simulink library "acolibjan22"  (R2021a)
settings: Solver=VariableStepAuto  StartTime=0.0  StopTime=10.0  RelTol=1e-3
libraries: simulink_extras x5, simulink x2, $bdroot x2
settings Model: Creator=e102261  LastModifiedBy=e102261
settings SolverCC: AlgebraicLoopSolver=TrustRegion
settings DebuggingCC: ArithmeticOperatorsInVariantConditions=warning
settings SFSimCC: CustomCodeUndefinedFunction=UseInterfaceOnly

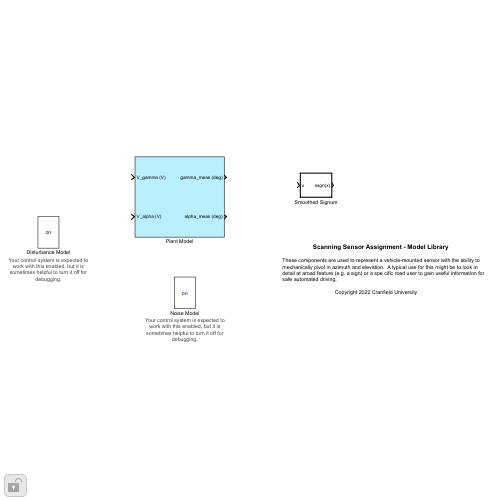
[thumbnail: Simulink's stored preview of the top-level diagram]
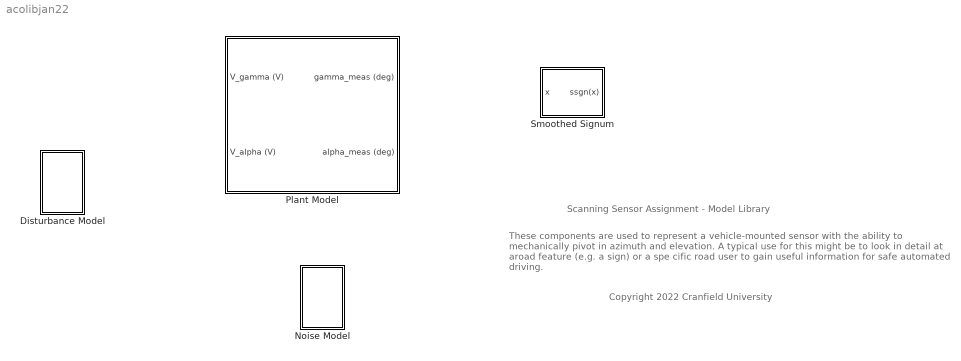
== system acolibjan22 ==
  note: Copyright 2022 Cranfield University
  note: Scanning Sensor Assignment - Model Library
  note: These components are used to represent a vehicle-mounted sensor with the ability to mechanically pivot in azimuth and elevation.  A typical use for this might be to look in
      | detail at aroad feature (e.g. a sign) or a spe cific road user to gain useful information for
      | safe automated driving.
  Disturbance Model : Subsystem  mask(Disturbance Model){EnabledState=on}
      mask prompts: EnabledState "Enable"
      mask help: This block implements a disturbance model.
      mask init:
      | if EnabledState
      |     theText = 'on';
      |     theColor = 'blue';
      | else
      |     theText = 'off';
      |     theColor = 'red';
      | end
      settings: AttributesFormatString=|
      | Your control system is expected to
      | work with this enabled, but it is
      | sometimes helpful to turn it off for
      | debugging.
      mask Display:
      | color(theColor);
      | fprintf(theText);
  Noise Model : Subsystem  mask(Noise Model){EnabledState=on}
      mask prompts: EnabledState "Enable"
      mask help: This block implements a noise model.
      mask init:
      | if EnabledState
      |     theText = 'on';
      |     theColor = 'blue';
      | else
      |     theText = 'off';
      |     theColor = 'red';
      | end
      settings: AttributesFormatString=|
      | Your control system is expected to
      | work with this enabled, but it is
      | sometimes helpful to turn it off for
      | debugging.
      mask Display:
      | color(theColor);
      | fprintf(theText);
  Plant Model : Subsystem  mask{X0=0}
      mask prompts: X0 "Initial state:"
      mask init:
      | if isequal(X0, 0)
      |     X0 = zeros(6,1);
      | else
      |     X0 = [X0(1); X0(2); X0(3); X0(4); X0(5); X0(6)];
      | end
  Smoothed Signum : Subsystem  TreatAsAtomicUnit=on  mask(Smoothed Signum){ApproxTransitionBand=0.1}
      mask prompts: ApproxTransitionBand "Approx. transition band (units):"
      mask help: This block implements a smoothed signum function, suitable for modelling stuff like friction. This can make it easier to implement near-hybrid models that execute nicely.
      mask init:
      | G = 1 / double(ApproxTransitionBand(1));

== system acolibjan22/Disturbance Model ==
  Constant : Constant  Value=EnabledState
  Enabled Subsystem : Subsystem
  tag scope: daz=global, del=global
  wires:
  Enabled Subsystem/1(daz) -> [daz]
  Enabled Subsystem/2(del) -> [del]
  Constant/1 -> Enabled Subsystem/Enable

== system acolibjan22/Noise Model ==
  Constant : Constant  Value=EnabledState
  Enabled Subsystem : Subsystem
  tag scope: waz=global, wel=global
  wires:
  Constant/1 -> Enabled Subsystem/Enable
  Enabled Subsystem/2(wel) -> [wel]
  Enabled Subsystem/1(waz) -> [waz]

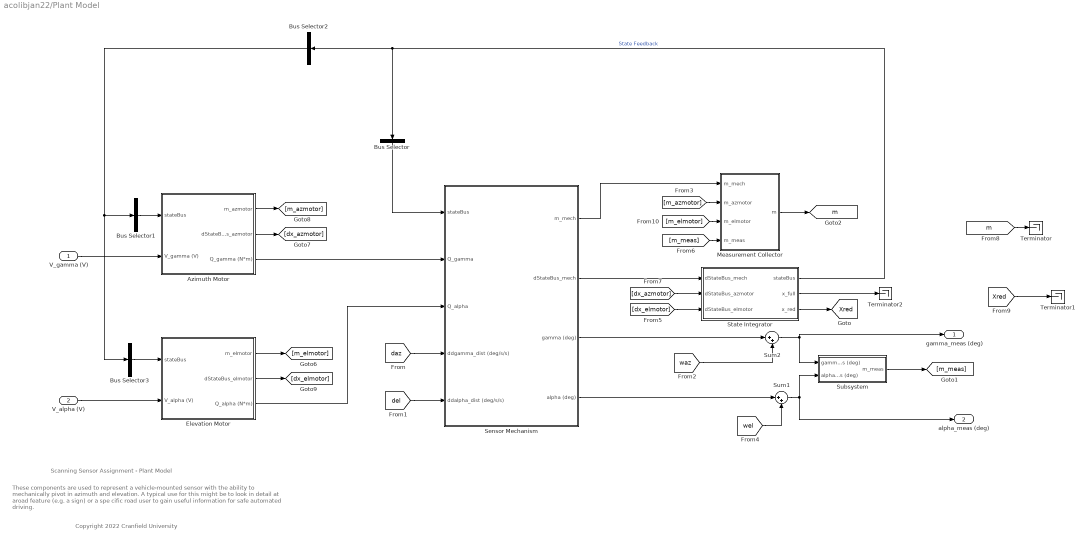
== system acolibjan22/Plant Model ==
  note: These components are used to represent a vehicle-mounted sensor with the ability to mechanically pivot in azimuth and elevation.  A typical use for this might be to look in
      | detail at aroad feature (e.g. a sign) or a spe cific road user to gain useful information for
      | safe automated driving.
  note: Scanning Sensor Assignment - Plant Model
  note: Copyright 2022 Cranfield University
  V_gamma (V) : Inport
  V_alpha (V) : Inport  Port=2
  Azimuth Motor : Subsystem
  Bus Selector : BusSelector  OutputSignals=gamma,dgamma,alpha,dalpha  OutputAsBus=on
  Bus Selector1 : BusSelector  OutputSignals=Q_gamma  OutputAsBus=on
  Bus Selector2 : BusSelector  OutputSignals=Q_gamma,Q_alpha  OutputAsBus=on
  Bus Selector3 : BusSelector  OutputSignals=Q_alpha  OutputAsBus=on
  Elevation Motor : Subsystem
  Measurement Collector : Subsystem
  Sensor Mechanism : Subsystem
  State Integrator : Subsystem
  Subsystem : Subsystem
  Sum1 : Sum  Inputs=|++
  Sum2 : Sum  Inputs=|++
  Terminator : Terminator
  Terminator1 : Terminator
  Terminator2 : Terminator
  gamma_meas (deg) : Outport
  alpha_meas (deg) : Outport  Port=2
  tag scope: Xred=global, m=global
  wires:
  [Xred] -> Terminator1/1
  Sensor Mechanism/4(alpha (deg)) -> Sum1/1
  Azimuth Motor/3(Q_gamma (N*m)) -> Sensor Mechanism/2(Q_gamma)
  V_gamma (V)/1 -> Azimuth Motor/2(V_gamma (V))
  [daz] -> Sensor Mechanism/4(ddgamma_dist (deg/s/s))
  [del] -> Sensor Mechanism/5(ddalpha_dist (deg/s/s))
  V_alpha (V)/1 -> Elevation Motor/2(V_alpha (V))
  State Integrator/1(stateBus) -> Bus Selector/1, Bus Selector2/1  "State Feedback"
  Azimuth Motor/1(m_azmotor) -> [m_azmotor]
  Measurement Collector/1(m) -> [m]
  [m_azmotor] -> Measurement Collector/2(m_azmotor)
  Azimuth Motor/2(dStateBus_azmotor) -> [dx_azmotor]
  [dx_azmotor] -> State Integrator/2(dStateBus_azmotor)
  Elevation Motor/1(m_elmotor) -> [m_elmotor]
  Elevation Motor/2(dStateBus_elmotor) -> [dx_elmotor]
  Elevation Motor/3(Q_alpha (N*m)) -> Sensor Mechanism/3(Q_alpha)
  [dx_elmotor] -> State Integrator/3(dStateBus_elmotor)
  [m_elmotor] -> Measurement Collector/3(m_elmotor)
  Sensor Mechanism/2(dStateBus_mech) -> State Integrator/1(dStateBus_mech)
  Sensor Mechanism/1(m_mech) -> Measurement Collector/1(m_mech)
  Bus Selector/1 -> Sensor Mechanism/1(stateBus)
  Bus Selector2/1 -> Bus Selector3/1, Bus Selector1/1
  Bus Selector1/1 -> Azimuth Motor/1(stateBus)
  Bus Selector3/1 -> Elevation Motor/1(stateBus)
  State Integrator/2(x_full) -> Terminator2/1
  State Integrator/3(x_red) -> [Xred]
  Sum1/1 -> Subsystem/2(alpha_meas (deg)), alpha_meas (deg)/1
  [wel] -> Sum1/2
  Sensor Mechanism/3(gamma (deg)) -> Sum2/1
  [waz] -> Sum2/2
  Sum2/1 -> Subsystem/1(gamma_meas (deg)), gamma_meas (deg)/1
  Subsystem/1(m_meas) -> [m_meas]
  [m_meas] -> Measurement Collector/4(m_meas)
  [m] -> Terminator/1

== system acolibjan22/Smoothed Signum ==
  x : Inport  PortDimensions=1
  Abs : Abs
  Product : Product  Inputs=3
  Product1 : Product
  Sign : Signum
  Transition Rate : Gain  Gain=8*G
  Trigonometric Function : Trigonometry  Operator=tanh
  ssgn(x) : Outport  PortDimensions=1
  wires:
  Product1/1 -> ssgn(x)/1
  Transition Rate/1 -> Trigonometric Function/1
  x/1 -> Sign/1, Transition Rate/1
  Trigonometric Function/1 -> Abs/1
  Abs/1 -> Product/3, Product/1, Product/2
  Product/1 -> Product1/1
  Sign/1 -> Product1/2

== system acolibjan22/Disturbance Model/Enabled Subsystem ==
  Enable : EnablePort
  Band-Limited White Noise : simulink/Sources/Band-Limited White Noise  Cov=5^2  Ts=0.8  seed=12414
  Band-Limited White Noise1 : simulink/Sources/Band-Limited White Noise  Cov=5^2  Ts=1.2  seed=43214517
  daz : Outport  OutputWhenDisabled=reset  InitialOutput=0
  del : Outport  Port=2  OutputWhenDisabled=reset  InitialOutput=0
  wires:
  Band-Limited White Noise1/1 -> del/1
  Band-Limited White Noise/1 -> daz/1

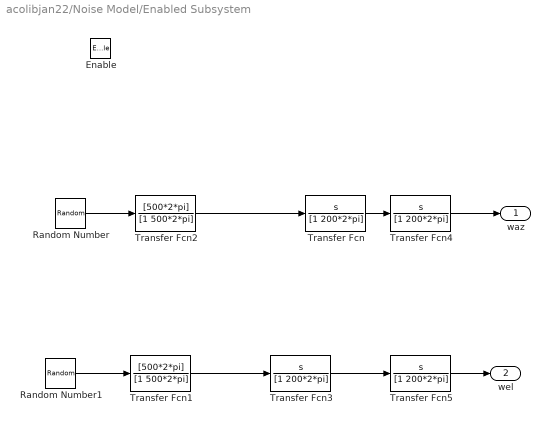
== system acolibjan22/Noise Model/Enabled Subsystem ==
  Enable : EnablePort
  Random Number : RandomNumber  Seed=8576  SampleTime=1/1000
  Random Number1 : RandomNumber  Seed=325325  SampleTime=1/500
  Transfer Fcn{,3..5} (4 alike) : TransferFcn  Numerator=[1 0]  Denominator=[1 200*2*pi]
  Transfer Fcn1 : TransferFcn  Numerator=[500*2*pi]  Denominator=[1 500*2*pi]
  Transfer Fcn2 : TransferFcn  Numerator=[500*2*pi]  Denominator=[1 500*2*pi]
  waz : Outport  OutputWhenDisabled=reset  InitialOutput=0
  wel : Outport  Port=2  OutputWhenDisabled=reset  InitialOutput=0
  wires:
  Transfer Fcn5/1 -> wel/1
  Transfer Fcn4/1 -> waz/1
  Transfer Fcn/1 -> Transfer Fcn4/1
  Random Number/1 -> Transfer Fcn2/1
  Transfer Fcn2/1 -> Transfer Fcn/1
  Random Number1/1 -> Transfer Fcn1/1
  Transfer Fcn3/1 -> Transfer Fcn5/1
  Transfer Fcn1/1 -> Transfer Fcn3/1

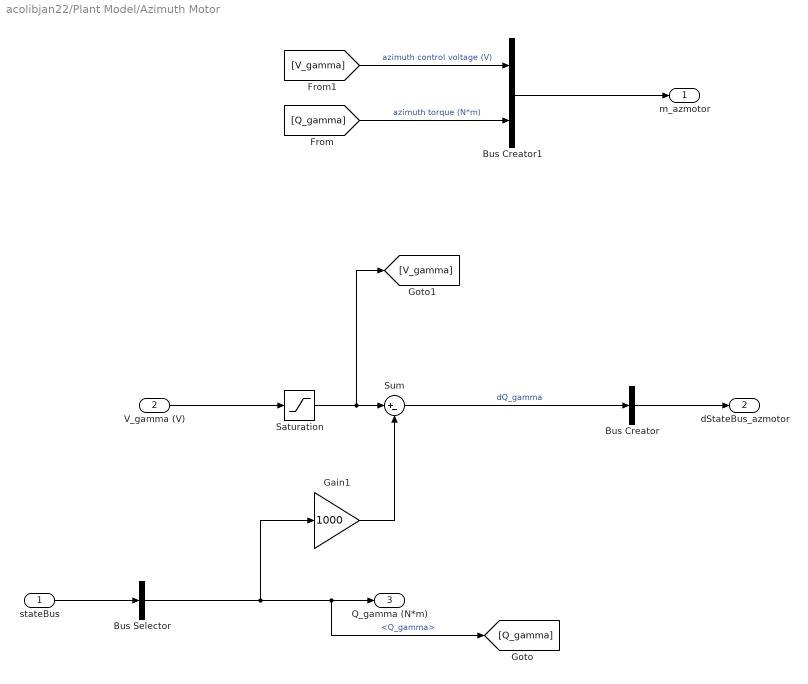
== system acolibjan22/Plant Model/Azimuth Motor ==
  stateBus : Inport
  V_gamma (V) : Inport  Port=2
  Bus Creator : BusCreator  Inputs=1
  Bus Creator1 : BusCreator  Inputs=2
  Bus Selector : BusSelector  OutputSignals=Q_gamma
  Gain1 : Gain  Gain=1000
  Saturation : Saturate  UpperLimit=+15  LowerLimit=-15
      settings: AttributesFormatString=|
      | UpperLimit=%<UpperLimit>
      | LowerLimit=%<LowerLimit>
  Sum : Sum  Inputs=|+-
  m_azmotor : Outport
  dStateBus_azmotor : Outport  Port=2
  Q_gamma (N*m) : Outport  Port=3
  wires:
  Saturation/1 -> [V_gamma], Sum/1
  V_gamma (V)/1 -> Saturation/1
  Gain1/1 -> Sum/2
  Sum/1 -> Bus Creator/1  "dQ_gamma"
  stateBus/1 -> Bus Selector/1
  Bus Selector/1 -> Gain1/1, [Q_gamma], Q_gamma (N*m)/1  "<Q_gamma>"
  Bus Creator/1 -> dStateBus_azmotor/1
  [Q_gamma] -> Bus Creator1/2  "azimuth torque (N*m)"
  [V_gamma] -> Bus Creator1/1  "azimuth control voltage (V)"
  Bus Creator1/1 -> m_azmotor/1

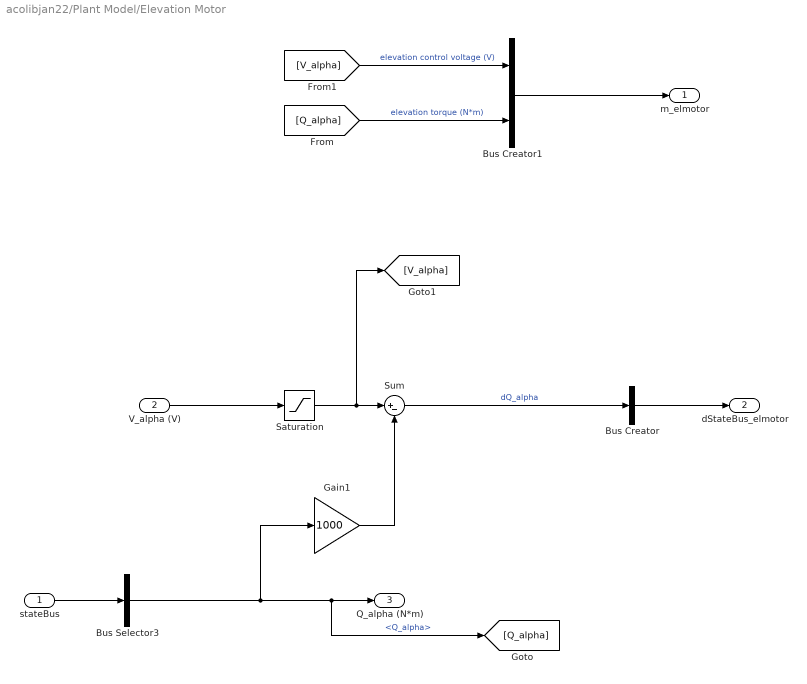
== system acolibjan22/Plant Model/Elevation Motor ==
  stateBus : Inport
  V_alpha (V) : Inport  Port=2
  Bus Creator : BusCreator  Inputs=1
  Bus Creator1 : BusCreator  Inputs=2
  Bus Selector3 : BusSelector  OutputSignals=Q_alpha
  Gain1 : Gain  Gain=1000
  Saturation : Saturate  UpperLimit=+15  LowerLimit=-15
      settings: AttributesFormatString=|
      | UpperLimit=%<UpperLimit>
      | LowerLimit=%<LowerLimit>
  Sum : Sum  Inputs=|+-
  m_elmotor : Outport
  dStateBus_elmotor : Outport  Port=2
  Q_alpha (N*m) : Outport  Port=3
  wires:
  Saturation/1 -> [V_alpha], Sum/1
  V_alpha (V)/1 -> Saturation/1
  Gain1/1 -> Sum/2
  Sum/1 -> Bus Creator/1  "dQ_alpha"
  stateBus/1 -> Bus Selector3/1
  Bus Creator/1 -> dStateBus_elmotor/1
  [Q_alpha] -> Bus Creator1/2  "elevation torque (N*m)"
  [V_alpha] -> Bus Creator1/1  "elevation control voltage (V)"
  Bus Creator1/1 -> m_elmotor/1
  Bus Selector3/1 -> Gain1/1, [Q_alpha], Q_alpha (N*m)/1  "<Q_alpha>"

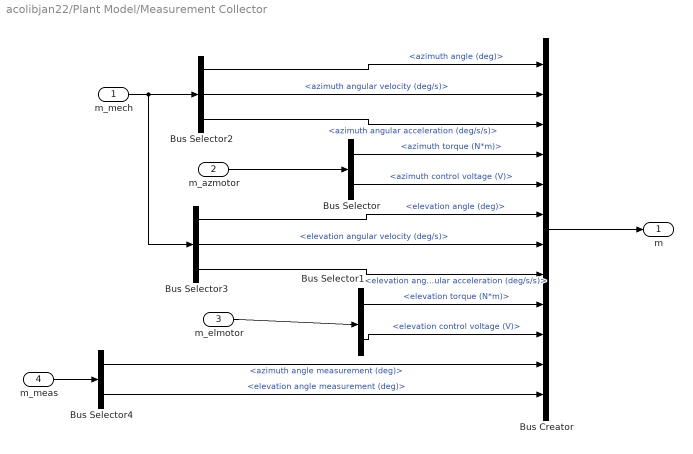
== system acolibjan22/Plant Model/Measurement Collector ==
  m_mech : Inport
  m_azmotor : Inport  Port=2
  m_elmotor : Inport  Port=3
  m_meas : Inport  Port=4
  Bus Creator : BusCreator  Inputs=12
  Bus Selector : BusSelector  OutputSignals=azimuth torque (N*m),azimuth control voltage (V)
  Bus Selector1 : BusSelector  OutputSignals=elevation torque (N*m),elevation control voltage (V)
  Bus Selector2 : BusSelector  OutputSignals=azimuth angle (deg),azimuth angular velocity (deg/s),azimuth angular acceleration (deg/s/s)
  Bus Selector3 : BusSelector  OutputSignals=elevation angle (deg),elevation angular velocity (deg/s),elevation angular acceleration (deg/s/s)
  Bus Selector4 : BusSelector  OutputSignals=azimuth angle measurement (deg),elevation angle measurement (deg)
  m : Outport
  wires:
  Bus Creator/1 -> m/1
  Bus Selector3/1 -> Bus Creator/6  "<elevation angle (deg)>"
  Bus Selector1/2 -> Bus Creator/10  "<elevation control voltage (V)>"
  Bus Selector1/1 -> Bus Creator/9  "<elevation torque (N*m)>"
  Bus Selector3/2 -> Bus Creator/7  "<elevation angular velocity (deg/s)>"
  Bus Selector3/3 -> Bus Creator/8  "<elevation angular acceleration (deg/s/s)>"
  m_azmotor/1 -> Bus Selector/1
  Bus Selector/1 -> Bus Creator/4  "<azimuth torque (N*m)>"
  Bus Selector/2 -> Bus Creator/5  "<azimuth control voltage (V)>"
  m_elmotor/1 -> Bus Selector1/1
  m_mech/1 -> Bus Selector3/1, Bus Selector2/1
  Bus Selector2/1 -> Bus Creator/1  "<azimuth angle (deg)>"
  Bus Selector2/2 -> Bus Creator/2  "<azimuth angular velocity (deg/s)>"
  Bus Selector2/3 -> Bus Creator/3  "<azimuth angular acceleration (deg/s/s)>"
  m_meas/1 -> Bus Selector4/1
  Bus Selector4/1 -> Bus Creator/11  "<azimuth angle measurement (deg)>"
  Bus Selector4/2 -> Bus Creator/12  "<elevation angle measurement (deg)>"

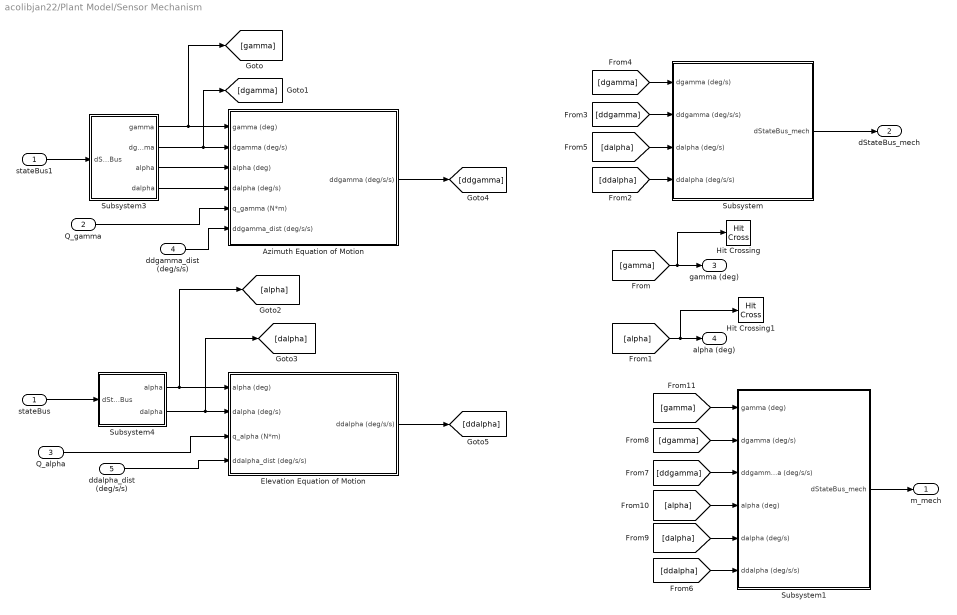
== system acolibjan22/Plant Model/Sensor Mechanism ==
  stateBus : Inport
  Q_gamma : Inport  Port=2
  Q_alpha : Inport  Port=3
  ddgamma_dist (deg/s/s) : Inport  Port=4
  ddalpha_dist (deg/s/s) : Inport  Port=5
  Azimuth Equation of Motion : Subsystem  mask{J=1e-3, Ja=0.020e-3, F=0.1e-3, k=1e-3}
      mask prompts: J "Fixed moment of inertia:"; Ja "Varying moment of inertia:"; F "Coefficient of friction (N*m):"; k "Coefficient of damping (N*m/rad/s):"
  Elevation Equation of Motion : Subsystem  mask(Elevation Dynamics){J=1e-3, F=0.1e-3, k=1e-3}
      mask prompts: J "Moment of inertia"; F "Coefficient of friction (N):"; k "Coefficient of damping (N*m/rad/s):"
      mask help: This block represents the elevantion dynamics of the sensor mount.
  Hit Crossing : HitCross  HitCrossingOffset=linspace(-180,180,361)  ShowOutputPort=off
  Hit Crossing1 : HitCross  HitCrossingOffset=linspace(-180,180,361)  ShowOutputPort=off
  Subsystem : Subsystem
  Subsystem1 : Subsystem
  Subsystem3 : Subsystem
  Subsystem4 : Subsystem
  stateBus1 : InportShadow
  m_mech : Outport
  dStateBus_mech : Outport  Port=2
  gamma (deg) : Outport  Port=3
  alpha (deg) : Outport  Port=4
  wires:
  ddalpha_dist (deg/s/s)/1 -> Elevation Equation of Motion/4(ddalpha_dist (deg/s/s))
  Elevation Equation of Motion/1(ddalpha (deg/s/s)) -> [ddalpha]
  ddgamma_dist (deg/s/s)/1 -> Azimuth Equation of Motion/6(ddgamma_dist (deg/s/s))
  Azimuth Equation of Motion/1(ddgamma (deg/s/s)) -> [ddgamma]
  stateBus1/1 -> Subsystem3/1(dStateBus)
  Q_gamma/1 -> Azimuth Equation of Motion/5(q_gamma (N*m))
  stateBus/1 -> Subsystem4/1(dStateBus)
  Q_alpha/1 -> Elevation Equation of Motion/3(q_alpha (N*m))
  Subsystem3/1(gamma) -> [gamma], Azimuth Equation of Motion/1(gamma (deg))
  Subsystem3/2(dgamma) -> [dgamma], Azimuth Equation of Motion/2(dgamma (deg/s))
  Subsystem3/3(alpha) -> Azimuth Equation of Motion/3(alpha (deg))
  Subsystem3/4(dalpha) -> Azimuth Equation of Motion/4(dalpha (deg/s))
  Subsystem4/1(alpha) -> Elevation Equation of Motion/1(alpha (deg)), [alpha]
  Subsystem4/2(dalpha) -> [dalpha], Elevation Equation of Motion/2(dalpha (deg/s))
  [gamma] -> Hit Crossing/1, gamma (deg)/1
  [alpha] -> Hit Crossing1/1, alpha (deg)/1
  [ddalpha] -> Subsystem/4(ddalpha (deg/s/s))
  [ddgamma] -> Subsystem/2(ddgamma (deg/s/s))
  [dgamma] -> Subsystem/1(dgamma (deg/s))
  [dalpha] -> Subsystem/3(dalpha (deg/s))
  Subsystem/1(dStateBus_mech) -> dStateBus_mech/1
  [ddalpha] -> Subsystem1/6(ddalpha (deg/s/s))
  [dalpha] -> Subsystem1/5(dalpha (deg/s))
  [ddgamma] -> Subsystem1/3(ddgamma (deg/s/s))
  [dgamma] -> Subsystem1/2(dgamma (deg/s))
  [alpha] -> Subsystem1/4(alpha (deg))
  [gamma] -> Subsystem1/1(gamma (deg))
  Subsystem1/1(dStateBus_mech) -> m_mech/1

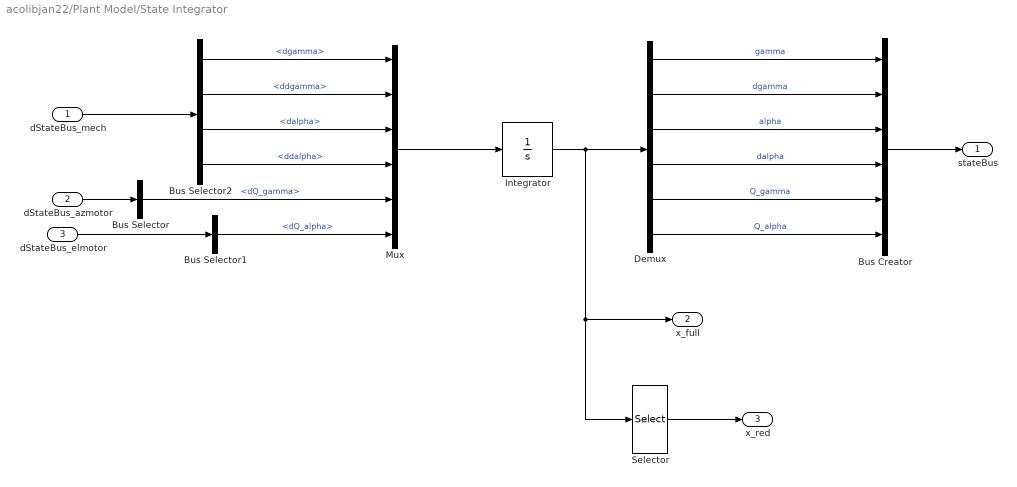
== system acolibjan22/Plant Model/State Integrator ==
  dStateBus_mech : Inport
  dStateBus_azmotor : Inport  Port=2
  dStateBus_elmotor : Inport  Port=3
  Bus Creator : BusCreator  Inputs=6
  Bus Selector : BusSelector  OutputSignals=dQ_gamma
  Bus Selector1 : BusSelector  OutputSignals=dQ_alpha
  Bus Selector2 : BusSelector  OutputSignals=dgamma,ddgamma,dalpha,ddalpha
  Demux : Demux  Outputs=6
  Integrator : Integrator  InitialCondition=X0
  Mux : Mux  Inputs=6
  Selector : Selector  InputPortWidth=6  IndexOptions=Index vector (dialog)  Indices=[1:4]  OutputSizes=1
  stateBus : Outport
  x_full : Outport  Port=2
  x_red : Outport  Port=3
  wires:
  Mux/1 -> Integrator/1
  Bus Selector/1 -> Mux/5  "<dQ_gamma>"
  dStateBus_azmotor/1 -> Bus Selector/1
  dStateBus_elmotor/1 -> Bus Selector1/1
  Bus Selector1/1 -> Mux/6  "<dQ_alpha>"
  dStateBus_mech/1 -> Bus Selector2/1
  Bus Selector2/1 -> Mux/1  "<dgamma>"
  Bus Selector2/2 -> Mux/2  "<ddgamma>"
  Bus Selector2/4 -> Mux/4  "<ddalpha>"
  Bus Selector2/3 -> Mux/3  "<dalpha>"
  Demux/3 -> Bus Creator/3  "alpha"
  Demux/6 -> Bus Creator/6  "Q_alpha"
  Demux/2 -> Bus Creator/2  "dgamma"
  Integrator/1 -> x_full/1, Selector/1, Demux/1
  Bus Creator/1 -> stateBus/1
  Demux/4 -> Bus Creator/4  "dalpha"
  Demux/5 -> Bus Creator/5  "Q_gamma"
  Demux/1 -> Bus Creator/1  "gamma"
  Selector/1 -> x_red/1

== system acolibjan22/Plant Model/Subsystem ==
  gamma_meas (deg) : Inport
  alpha_meas (deg) : Inport  Port=2
  Bus Creator : BusCreator  Inputs=2
  m_meas : Outport
  wires:
  gamma_meas (deg)/1 -> Bus Creator/1  "azimuth angle measurement (deg)"
  alpha_meas (deg)/1 -> Bus Creator/2  "elevation angle measurement (deg)"
  Bus Creator/1 -> m_meas/1

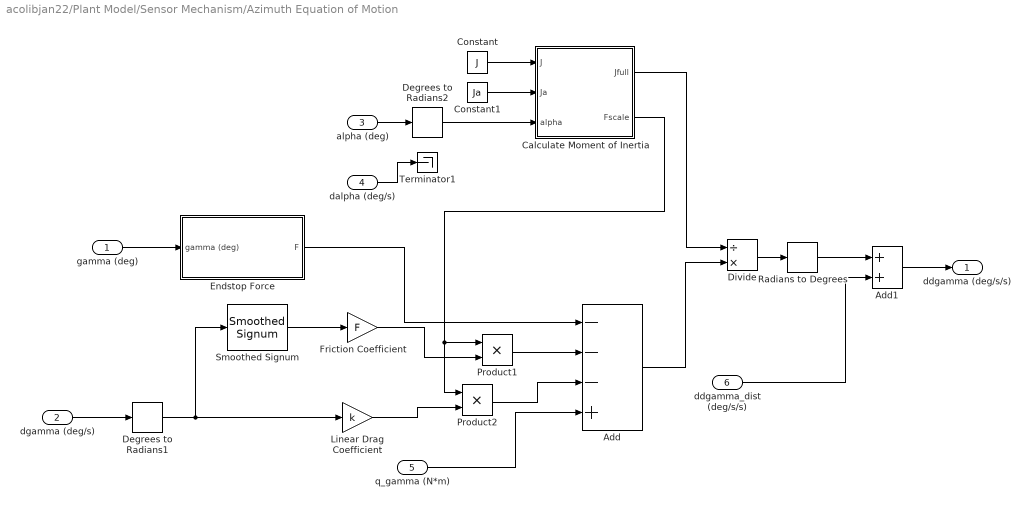
== system acolibjan22/Plant Model/Sensor Mechanism/Azimuth Equation of Motion ==
  gamma (deg) : Inport
  dgamma (deg/s) : Inport  Port=2
  alpha (deg) : Inport  Port=3
  dalpha (deg/s) : Inport  Port=4
  q_gamma (N*m) : Inport  Port=5
  ddgamma_dist (deg/s/s) : Inport  Port=6
  Add : Sum  Inputs=---+
  Add1 : Sum
  Calculate Moment of Inertia : Subsystem
  Constant : Constant  Value=J
  Constant1 : Constant  Value=Ja
  Degrees to Radians1 : simulink_extras/Transformations/Degrees to Radians
  Degrees to Radians2 : simulink_extras/Transformations/Degrees to Radians
  Divide : Product  Inputs=/*
  Endstop Force : Subsystem
  Friction Coefficient : Gain  Gain=F
  Linear Drag Coefficient : Gain  Gain=k
  Product1 : Product
  Product2 : Product
  Radians to Degrees : simulink_extras/Transformations/Radians to Degrees
  Smoothed Signum : $bdroot/Smoothed Signum  ApproxTransitionBand=0.1
  Terminator1 : Terminator
  ddgamma (deg/s/s) : Outport
  wires:
  Product2/1 -> Add/3
  Product1/1 -> Add/2
  Calculate Moment of Inertia/2(Fscale) -> Product2/1, Product1/1
  Radians to Degrees/1 -> Add1/1
  Add1/1 -> ddgamma (deg/s/s)/1
  ddgamma_dist (deg/s/s)/1 -> Add1/2
  Divide/1 -> Radians to Degrees/1
  Add/1 -> Divide/2
  Linear Drag Coefficient/1 -> Product2/2
  q_gamma (N*m)/1 -> Add/4
  Degrees to Radians1/1 -> Smoothed Signum/1, Linear Drag Coefficient/1
  dgamma (deg/s)/1 -> Degrees to Radians1/1
  Friction Coefficient/1 -> Product1/2
  Smoothed Signum/1 -> Friction Coefficient/1
  alpha (deg)/1 -> Degrees to Radians2/1
  Constant/1 -> Calculate Moment of Inertia/1(J)
  Degrees to Radians2/1 -> Calculate Moment of Inertia/3(alpha)
  Constant1/1 -> Calculate Moment of Inertia/2(Ja)
  Calculate Moment of Inertia/1(Jfull) -> Divide/1
  gamma (deg)/1 -> Endstop Force/1(gamma (deg))
  dalpha (deg/s)/1 -> Terminator1/1
  Endstop Force/1(F) -> Add/1

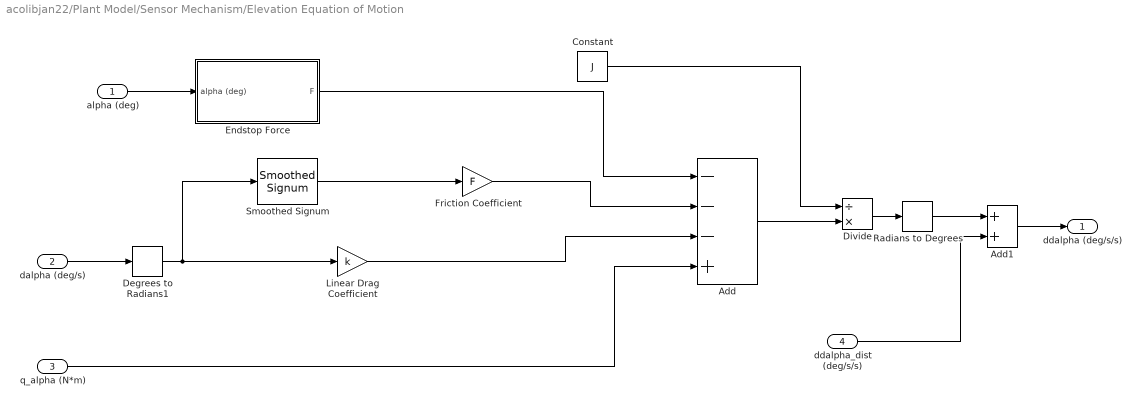
== system acolibjan22/Plant Model/Sensor Mechanism/Elevation Equation of Motion ==
  alpha (deg) : Inport
  dalpha (deg/s) : Inport  Port=2
  q_alpha (N*m) : Inport  Port=3
  ddalpha_dist (deg/s/s) : Inport  Port=4
  Add : Sum  Inputs=---+
  Add1 : Sum
  Constant : Constant  Value=J
  Degrees to Radians1 : simulink_extras/Transformations/Degrees to Radians
  Divide : Product  Inputs=/*
  Endstop Force : Subsystem
  Friction Coefficient : Gain  Gain=F
  Linear Drag Coefficient : Gain  Gain=k
  Radians to Degrees : simulink_extras/Transformations/Radians to Degrees
  Smoothed Signum : $bdroot/Smoothed Signum  ApproxTransitionBand=0.1
  ddalpha (deg/s/s) : Outport
  wires:
  Smoothed Signum/1 -> Friction Coefficient/1
  Friction Coefficient/1 -> Add/2
  dalpha (deg/s)/1 -> Degrees to Radians1/1
  Degrees to Radians1/1 -> Linear Drag Coefficient/1, Smoothed Signum/1
  q_alpha (N*m)/1 -> Add/4
  Linear Drag Coefficient/1 -> Add/3
  Add/1 -> Divide/2
  Divide/1 -> Radians to Degrees/1
  ddalpha_dist (deg/s/s)/1 -> Add1/2
  Add1/1 -> ddalpha (deg/s/s)/1
  Radians to Degrees/1 -> Add1/1
  Constant/1 -> Divide/1
  alpha (deg)/1 -> Endstop Force/1(alpha (deg))
  Endstop Force/1(F) -> Add/1

== system acolibjan22/Plant Model/Sensor Mechanism/Subsystem ==
  dgamma (deg/s) : Inport
  ddgamma (deg/s/s) : Inport  Port=2
  dalpha (deg/s) : Inport  Port=3
  ddalpha (deg/s/s) : Inport  Port=4
  Bus Creator : BusCreator  Inputs=4
  dStateBus_mech : Outport
  wires:
  ddgamma (deg/s/s)/1 -> Bus Creator/2  "ddgamma"
  dgamma (deg/s)/1 -> Bus Creator/1  "dgamma"
  Bus Creator/1 -> dStateBus_mech/1
  ddalpha (deg/s/s)/1 -> Bus Creator/4  "ddalpha"
  dalpha (deg/s)/1 -> Bus Creator/3  "dalpha"

== system acolibjan22/Plant Model/Sensor Mechanism/Subsystem1 ==
  gamma (deg) : Inport
  dgamma (deg/s) : Inport  Port=2
  ddgamma (deg/s/s) : Inport  Port=3
  alpha (deg) : Inport  Port=4
  dalpha (deg/s) : Inport  Port=5
  ddalpha (deg/s/s) : Inport  Port=6
  Bus Creator : BusCreator  Inputs=6
  dStateBus_mech : Outport
  wires:
  dalpha (deg/s)/1 -> Bus Creator/5  "elevation angular velocity (deg/s)"
  ddalpha (deg/s/s)/1 -> Bus Creator/6  "elevation angular acceleration (deg/s/s)"
  Bus Creator/1 -> dStateBus_mech/1
  dgamma (deg/s)/1 -> Bus Creator/2  "azimuth angular velocity (deg/s)"
  ddgamma (deg/s/s)/1 -> Bus Creator/3  "azimuth angular acceleration (deg/s/s)"
  alpha (deg)/1 -> Bus Creator/4  "elevation angle (deg)"
  gamma (deg)/1 -> Bus Creator/1  "azimuth angle (deg)"

== system acolibjan22/Plant Model/Sensor Mechanism/Subsystem3 ==
  dStateBus : Inport
  Bus Selector2 : BusSelector  OutputSignals=gamma,dgamma,alpha,dalpha
  gamma : Outport
  dgamma : Outport  Port=2
  alpha : Outport  Port=3
  dalpha : Outport  Port=4
  wires:
  Bus Selector2/4 -> dalpha/1  "<dalpha>"
  Bus Selector2/2 -> dgamma/1  "<dgamma>"
  Bus Selector2/3 -> alpha/1  "<alpha>"
  Bus Selector2/1 -> gamma/1  "<gamma>"
  dStateBus/1 -> Bus Selector2/1

== system acolibjan22/Plant Model/Sensor Mechanism/Subsystem4 ==
  dStateBus : Inport
  Bus Selector2 : BusSelector  OutputSignals=alpha,dalpha
  alpha : Outport
  dalpha : Outport  Port=2
  wires:
  dStateBus/1 -> Bus Selector2/1
  Bus Selector2/1 -> alpha/1  "<alpha>"
  Bus Selector2/2 -> dalpha/1  "<dalpha>"

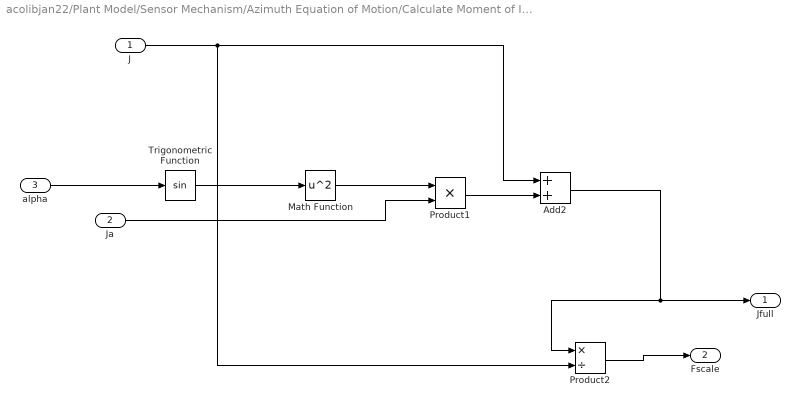
== system acolibjan22/Plant Model/Sensor Mechanism/Azimuth Equation of Motion/Calculate Moment of Inertia ==
  J : Inport
  Ja : Inport  Port=2
  alpha : Inport  Port=3
  Add2 : Sum
  Math Function : Math  Operator=square  SignedPower=on  SaturateOnIntegerOverflow=on
  Product1 : Product
  Product2 : Product  Inputs=*/
  Trigonometric Function : Trigonometry
  Jfull : Outport
  Fscale : Outport  Port=2
  wires:
  Product2/1 -> Fscale/1
  J/1 -> Add2/1, Product2/2
  Product1/1 -> Add2/2
  Trigonometric Function/1 -> Math Function/1
  Ja/1 -> Product1/2
  Math Function/1 -> Product1/1
  Add2/1 -> Product2/1, Jfull/1
  alpha/1 -> Trigonometric Function/1

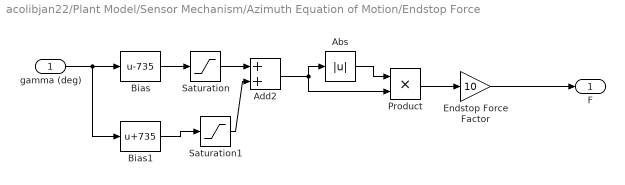
== system acolibjan22/Plant Model/Sensor Mechanism/Azimuth Equation of Motion/Endstop Force ==
  gamma (deg) : Inport
  Abs : Abs
  Add2 : Sum
  Bias : Bias  Bias=-735
  Bias1 : Bias  Bias=735
  Endstop Force Factor : Gain  Gain=10
  Product : Product
  Saturation : Saturate  UpperLimit=inf  LowerLimit=0
  Saturation1 : Saturate  UpperLimit=0  LowerLimit=-inf
  F : Outport
  wires:
  Bias/1 -> Saturation/1
  gamma (deg)/1 -> Bias1/1, Bias/1
  Saturation/1 -> Add2/1
  Add2/1 -> Product/2, Abs/1
  Abs/1 -> Product/1
  Endstop Force Factor/1 -> F/1
  Product/1 -> Endstop Force Factor/1
  Bias1/1 -> Saturation1/1
  Saturation1/1 -> Add2/2

== system acolibjan22/Plant Model/Sensor Mechanism/Elevation Equation of Motion/Endstop Force ==
  alpha (deg) : Inport
  Abs : Abs
  Add2 : Sum
  Bias : Bias  Bias=-75
  Bias1 : Bias  Bias=75
  Endstop Force Factor : Gain  Gain=10
  Product : Product
  Saturation : Saturate  UpperLimit=inf  LowerLimit=0
  Saturation1 : Saturate  UpperLimit=0  LowerLimit=-inf
  F : Outport
  wires:
  Bias/1 -> Saturation/1
  alpha (deg)/1 -> Bias1/1, Bias/1
  Saturation/1 -> Add2/1
  Add2/1 -> Product/2, Abs/1
  Abs/1 -> Product/1
  Endstop Force Factor/1 -> F/1
  Product/1 -> Endstop Force Factor/1
  Bias1/1 -> Saturation1/1
  Saturation1/1 -> Add2/2
